simulink model "model"  (R2020b)
settings: Solver=VariableStepAuto  StartTime=0.0  StopTime=1  RelTol=1e-3
undefined symbols (not defined in the file): B, flux, J, L, P, Rs, trap, Ts
settings Model: Creator=Lenovo  LastModifiedBy=Lenovo

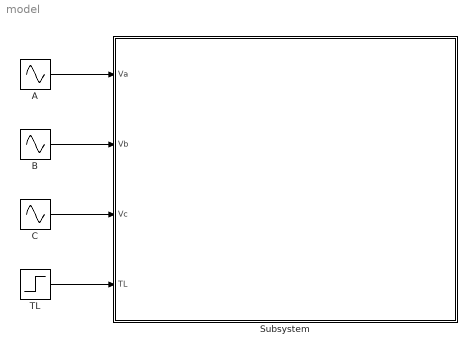
== system model ==
  A : Sin  Amplitude=220*sqrt(2)  Frequency=2*pi*50  SampleTime=Ts
  B : Sin  Amplitude=220*sqrt(2)  Frequency=2*pi*50  Phase=-2*pi/3  SampleTime=Ts
  C : Sin  Amplitude=220*sqrt(2)  Frequency=2*pi*50  Phase=2*pi/3  SampleTime=Ts
  Subsystem : Subsystem
  TL : Step  Time=0.5  After=10  SampleTime=0
  wires:
  TL/1 -> Subsystem/4(TL)
  C/1 -> Subsystem/3(Vc)
  B/1 -> Subsystem/2(Vb)
  A/1 -> Subsystem/1(Va)

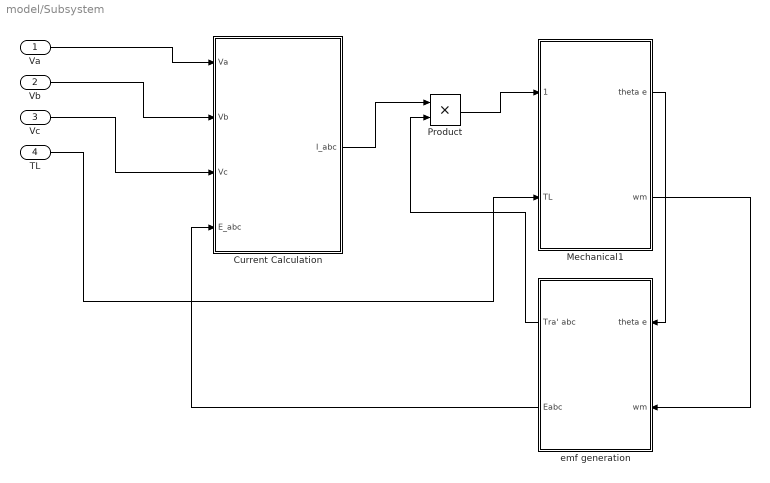
== system model/Subsystem ==
  Va : Inport
  Vb : Inport  Port=2
  Vc : Inport  Port=3
  TL : Inport  Port=4
  Current Calculation : Subsystem
  Mechanical1 : Subsystem
  Product : Product
  emf generation : Subsystem
  wires:
  Va/1 -> Current Calculation/1(Va)
  Vb/1 -> Current Calculation/2(Vb)
  emf generation/2(Eabc) -> Current Calculation/4(E_abc)
  Vc/1 -> Current Calculation/3(Vc)
  emf generation/1(Tra' abc) -> Product/2
  Mechanical1/2(wm) -> emf generation/2(wm)
  Product/1 -> Mechanical1/1(1)
  TL/1 -> Mechanical1/2(TL)
  Mechanical1/1(theta e) -> emf generation/1(theta e)
  Current Calculation/1(I_abc) -> Product/1

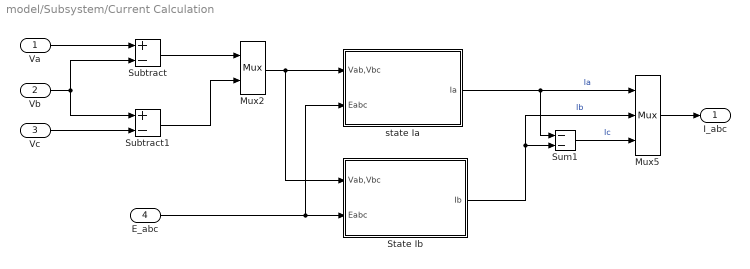
== system model/Subsystem/Current Calculation ==
  Va : Inport
  Vb : Inport  Port=2
  Vc : Inport  Port=3
  E_abc : Inport  Port=4
  Mux2 : Mux  Inputs=2
      settings: DisplayOption=signals
  Mux5 : Mux  Inputs=3
      settings: DisplayOption=signals
  State Ib : Subsystem
  Subtract : Sum  Inputs=+-
  Subtract1 : Sum  Inputs=+-
  Sum1 : Sum  Inputs=--  SaturateOnIntegerOverflow=on
  state Ia : Subsystem
  I_abc : Outport
  wires:
  State Ib/1(Ib) -> Sum1/2, Mux5/2  "Ib"
  Subtract1/1 -> Mux2/2
  Subtract/1 -> Mux2/1
  Vc/1 -> Subtract1/2
  Vb/1 -> Subtract1/1, Subtract/2
  Va/1 -> Subtract/1
  state Ia/1(Ia) -> Mux5/1, Sum1/1  "Ia"
  Sum1/1 -> Mux5/3  "Ic"
  Mux5/1 -> I_abc/1
  Mux2/1 -> State Ib/1(Vab,Vbc), state Ia/1(Vab,Vbc)
  E_abc/1 -> State Ib/2(Eabc), state Ia/2(Eabc)

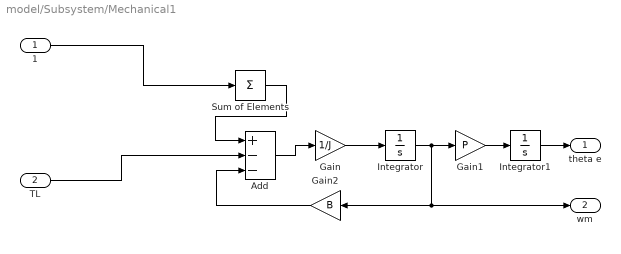
== system model/Subsystem/Mechanical1 ==
  1 : Inport
  TL : Inport  Port=2
  Add : Sum  Inputs=+--
  Gain : Gain  Gain=1/J
  Gain1 : Gain  Gain=P
  Gain2 : Gain  Gain=B
  Integrator : Integrator
  Integrator1 : Integrator
  Sum of Elements : Sum  Inputs=+
  theta e : Outport
  wm : Outport  Port=2
  wires:
  Integrator/1 -> Gain2/1, wm/1, Gain1/1
  Add/1 -> Gain/1
  Gain/1 -> Integrator/1
  Gain1/1 -> Integrator1/1
  1/1 -> Sum of Elements/1
  Sum of Elements/1 -> Add/1
  TL/1 -> Add/2
  Gain2/1 -> Add/3
  Integrator1/1 -> theta e/1

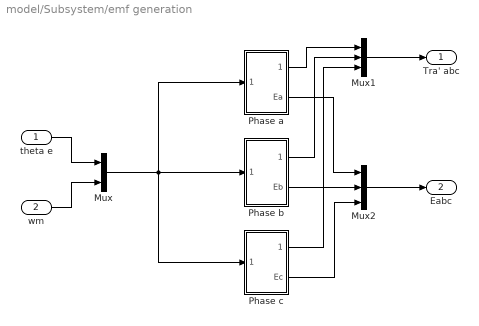
== system model/Subsystem/emf generation ==
  theta e : Inport
  wm : Inport  Port=2
  Mux : Mux  Inputs=2
  Mux1 : Mux  Inputs=3
  Mux2 : Mux  Inputs=3
  Phase a : Subsystem
  Phase b : Subsystem
  Phase c : Subsystem
  Tra' abc : Outport
  Eabc : Outport  Port=2
  wires:
  wm/1 -> Mux/2
  theta e/1 -> Mux/1
  Mux/1 -> Phase a/1(In1), Phase c/1(In1), Phase b/1(In1)
  Phase c/2(Ec) -> Mux2/3
  Mux1/1 -> Tra' abc/1
  Phase a/1(Tra' a) -> Mux1/1
  Phase c/1(Tra' c) -> Mux1/3
  Phase b/1(Tra' b) -> Mux1/2
  Phase b/2(Eb) -> Mux2/2
  Phase a/2(Ea) -> Mux2/1
  Mux2/1 -> Eabc/1

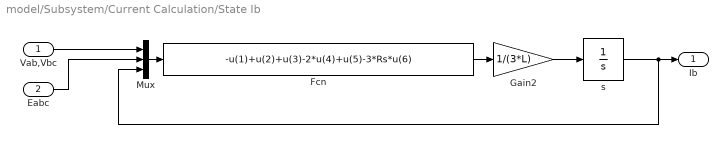
== system model/Subsystem/Current Calculation/State Ib ==
  Vab,Vbc : Inport
  Eabc : Inport  Port=2
  Fcn : Fcn  Expr=-u(1)+u(2)+u(3)-2*u(4)+u(5)-3*Rs*u(6)
  Gain2 : Gain  Gain=1/(3*L)  SaturateOnIntegerOverflow=on  OutDataTypeStr=Inherit: Same as input  ParamDataTypeStr=Inherit: Same as input
  Mux : Mux  Inputs=3
  "s " : Integrator
  Ib : Outport
  wires:
  "s "/1 -> Ib/1, Mux/3
  Fcn/1 -> Gain2/1
  Mux/1 -> Fcn/1
  Eabc/1 -> Mux/2
  Vab,Vbc/1 -> Mux/1
  Gain2/1 -> "s "/1

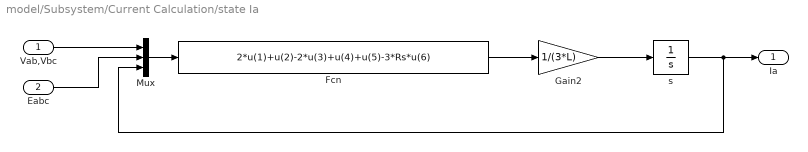
== system model/Subsystem/Current Calculation/state Ia ==
  Vab,Vbc : Inport
  Eabc : Inport  Port=2
  Fcn : Fcn  Expr=2*u(1)+u(2)-2*u(3)+u(4)+u(5)-3*Rs*u(6)
  Gain2 : Gain  Gain=1/(3*L)  SaturateOnIntegerOverflow=on  OutDataTypeStr=Inherit: Same as input  ParamDataTypeStr=Inherit: Same as input
  Mux : Mux  Inputs=3
  "s " : Integrator
  Ia : Outport
  wires:
  Gain2/1 -> "s "/1
  Vab,Vbc/1 -> Mux/1
  Eabc/1 -> Mux/2
  Mux/1 -> Fcn/1
  Fcn/1 -> Gain2/1
  "s "/1 -> Ia/1, Mux/3

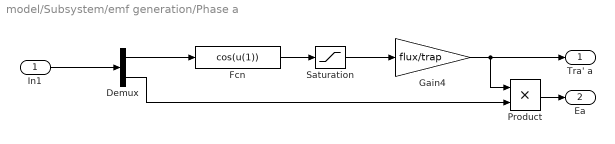
== system model/Subsystem/emf generation/Phase a ==
  In1 : Inport
  Demux : Demux  Outputs=2
  Fcn : Fcn  Expr=cos(u(1))
  Gain4 : Gain  Gain=flux/trap  SaturateOnIntegerOverflow=on  OutDataTypeStr=Inherit: Same as input  ParamDataTypeStr=Inherit: Same as input
  Product : Product
  Saturation : Saturate  UpperLimit=trap  LowerLimit=-trap
  Tra' a : Outport
  Ea : Outport  Port=2
  wires:
  Product/1 -> Ea/1
  In1/1 -> Demux/1
  Demux/2 -> Product/2
  Demux/1 -> Fcn/1
  Gain4/1 -> Tra' a/1, Product/1
  Saturation/1 -> Gain4/1
  Fcn/1 -> Saturation/1

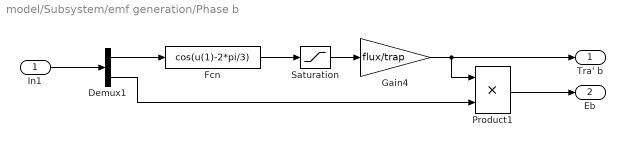
== system model/Subsystem/emf generation/Phase b ==
  In1 : Inport
  Demux1 : Demux  Outputs=2
  Fcn : Fcn  Expr=cos(u(1)-2*pi/3)
  Gain4 : Gain  Gain=flux/trap  SaturateOnIntegerOverflow=on  OutDataTypeStr=Inherit: Same as input  ParamDataTypeStr=Inherit: Same as input
  Product1 : Product  SaturateOnIntegerOverflow=on  OutDataTypeStr=Inherit: Same as first input
  Saturation : Saturate  UpperLimit=trap  LowerLimit=-trap
  Tra' b : Outport
  Eb : Outport  Port=2
  wires:
  Demux1/1 -> Fcn/1
  Product1/1 -> Eb/1
  In1/1 -> Demux1/1
  Gain4/1 -> Tra' b/1, Product1/1
  Demux1/2 -> Product1/2
  Fcn/1 -> Saturation/1
  Saturation/1 -> Gain4/1

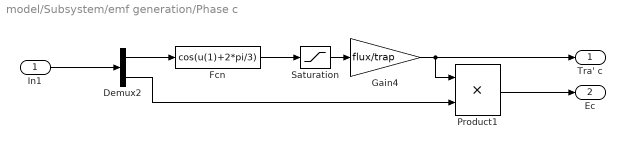
== system model/Subsystem/emf generation/Phase c ==
  In1 : Inport
  Demux2 : Demux  Outputs=2
  Fcn : Fcn  Expr=cos(u(1)+2*pi/3)
  Gain4 : Gain  Gain=flux/trap  SaturateOnIntegerOverflow=on  OutDataTypeStr=Inherit: Same as input  ParamDataTypeStr=Inherit: Same as input
  Product1 : Product  SaturateOnIntegerOverflow=on  OutDataTypeStr=Inherit: Same as first input
  Saturation : Saturate  UpperLimit=trap  LowerLimit=-trap
  Tra' c : Outport
  Ec : Outport  Port=2
  wires:
  In1/1 -> Demux2/1
  Gain4/1 -> Tra' c/1, Product1/1
  Fcn/1 -> Saturation/1
  Demux2/2 -> Product1/2
  Saturation/1 -> Gain4/1
  Product1/1 -> Ec/1
  Demux2/1 -> Fcn/1
